simulink model "rm3_ckt_DD_gen_vR2021b"  (R2021b)
settings: Solver=ode4  StartTime=0.0  StopTime=simu.duration  FixedStep=simu.timestep  MaxStep=0.1  MinStep=0.1  RelTol=1e-3
undefined symbols (not defined in the file or in its folder): PTO, R_pto
libraries: fl_lib x22, nesl_utility x19, ee_lib x14
settings Model: Creator=tedbrekken  LastModifiedBy=prana

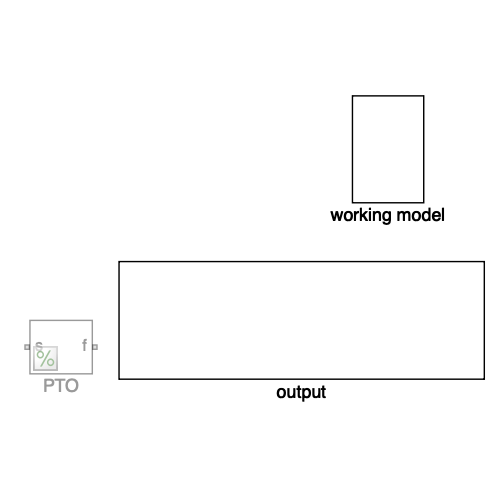
[thumbnail: Simulink's stored preview of the top-level diagram]
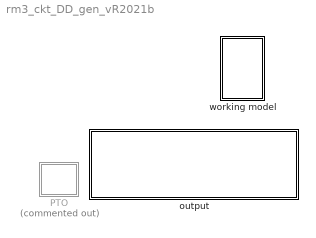
== system rm3_ckt_DD_gen_vR2021b ==
  PTO : Subsystem  Commented=on
  output : Subsystem
  working model : Subsystem

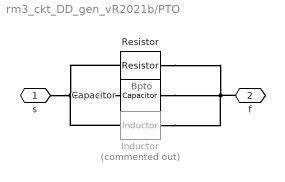
== system rm3_ckt_DD_gen_vR2021b/PTO ==
  note: Bpto
  Capacitor : fl_lib/Electrical/Electrical Elements/Capacitor  c=C_pto F  r=1e-6 Ohm  g=0 1/Ohm  i_specify=off  i_priority=None  i=0 A  i_nominal_specify=off  i_nominal_unit=A  i_nominal_value=1  v_specify=off  v_priority=None  v=0 V  v_nominal_specify=off  v_nominal_unit=V  v_nominal_value=1  vc_specify=off  vc_priority=High  vc=0 V  vc_nominal_specify=off  vc_nominal_unit=V  vc_nominal_value=1
  Inductor : ee_lib/Passive/Inductor  Commented=on  l=L_pto H  L_tol=20  enable_L_tol=0  tol_distribution=1  nSigma=4  r=0 Ohm  g=1e-9 1/Ohm  enable_operating_limits=0  operating_limit_action=2  max_working_current=1 A  power_rating=1 W  enable_faults=0  fault_action=1  lambdaPercent=50  k_faulted=0.9999  turnsShort=0  openCct=0  groundShort=0  groundShortG=0 1/Ohm  tau_fault=1e-3 s  enable_temporal_fault=0  t_fault=1 s  enable_behavioral_fault=0  max_permissible_voltage=100 V  n_fail_on_voltage=1  max_permissible_current=1 A  t_fail_on_current=1 s  i_L_specify=off  i_L_priority=High  i_L=0 A  i_L_nominal_specify=off  i_L_nominal_unit=A  i_L_nominal_value=1
  Resistor : ee_lib/Passive/Resistor  R=R_pto Ohm  R_tol=5  enable_R_tol=0  tol_distribution=1  nSigma=4  enable_operating_limits=0  operating_limit_action=2  max_working_voltage=100 V  power_rating=1 W  enable_faults=0  fault_action=1  R_faulted=inf Ohm  enable_temporal_fault=0  t_fault=1 s  enable_behavioral_fault=0  max_permissible_current=1 A  t_fail_on_current=1 s  noise_mode=0  sample_time=1e-3 s  repeatability=1  auto_seed=3499211588  user_seed=0  Tdevice=25 degC  power_derating_T1=70 degC  power_derating_T2=155 degC  operating_temperature_range_vec=[-50, 150] degC  alpha=3.93e-3 1/K  Tmeas=25 degC  thermal_mass=100 J/K  temperature_specify=off  temperature_priority=High  temperature=298.15 K  temperature_nominal_specify=off  temperature_nominal_unit=K  temperature_nominal_value=1
  s : PMIOPort  Side=Left
  f : PMIOPort  Port=2  Side=Right
  connections:
  s/RConn1 -- Resistor/LConn1 -- Inductor/LConn1 -- Capacitor/LConn1
  f/RConn1 -- Resistor/RConn1 -- Inductor/RConn1 -- Capacitor/RConn1

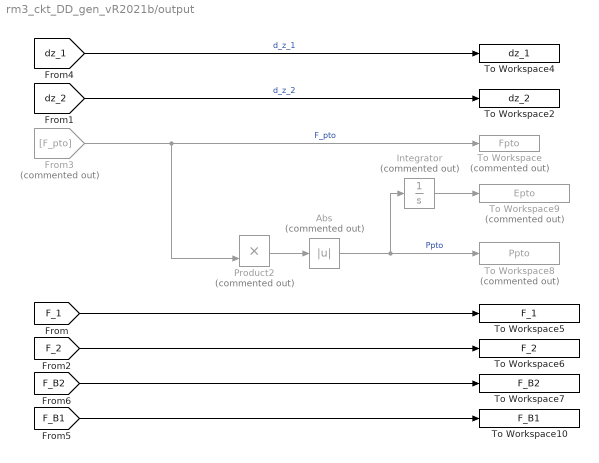
== system rm3_ckt_DD_gen_vR2021b/output ==
  Abs : Abs  Commented=on
  From3 : From  Commented=on  GotoTag=F_pto  TagVisibility=global
  Integrator : Integrator  Commented=on
  Product2 : Product  Commented=on
  To Workspace : ToWorkspace  Commented=on  VariableName=Fpto  SaveFormat=Timeseries  SampleTime=-1
  To Workspace10 : ToWorkspace  VariableName=F_B1  SaveFormat=Timeseries  SampleTime=-1
  To Workspace2 : ToWorkspace  VariableName=dz_2  SaveFormat=Timeseries  SampleTime=-1
  To Workspace4 : ToWorkspace  VariableName=dz_1  SaveFormat=Timeseries  SampleTime=-1
  To Workspace5 : ToWorkspace  VariableName=F_1  SaveFormat=Timeseries  SampleTime=-1
  To Workspace6 : ToWorkspace  VariableName=F_2  SaveFormat=Timeseries  SampleTime=-1
  To Workspace7 : ToWorkspace  VariableName=F_B2  SaveFormat=Timeseries  SampleTime=-1
  To Workspace8 : ToWorkspace  Commented=on  VariableName=Ppto  SaveFormat=Timeseries  SampleTime=-1
  To Workspace9 : ToWorkspace  Commented=on  VariableName=Epto  SaveFormat=Timeseries  SampleTime=-1
  wires:
  Integrator/1 -> To Workspace9/1
  [dz_1] -> To Workspace4/1  "d_z_1"
  From3/1 -> To Workspace/1, Product2/2  "F_pto"
  Abs/1 -> To Workspace8/1, Integrator/1  "Ppto"
  Product2/1 -> Abs/1
  [dz_2] -> To Workspace2/1  "d_z_2"
  [F_1] -> To Workspace5/1
  [F_2] -> To Workspace6/1
  [F_B2] -> To Workspace7/1
  [F_B1] -> To Workspace10/1

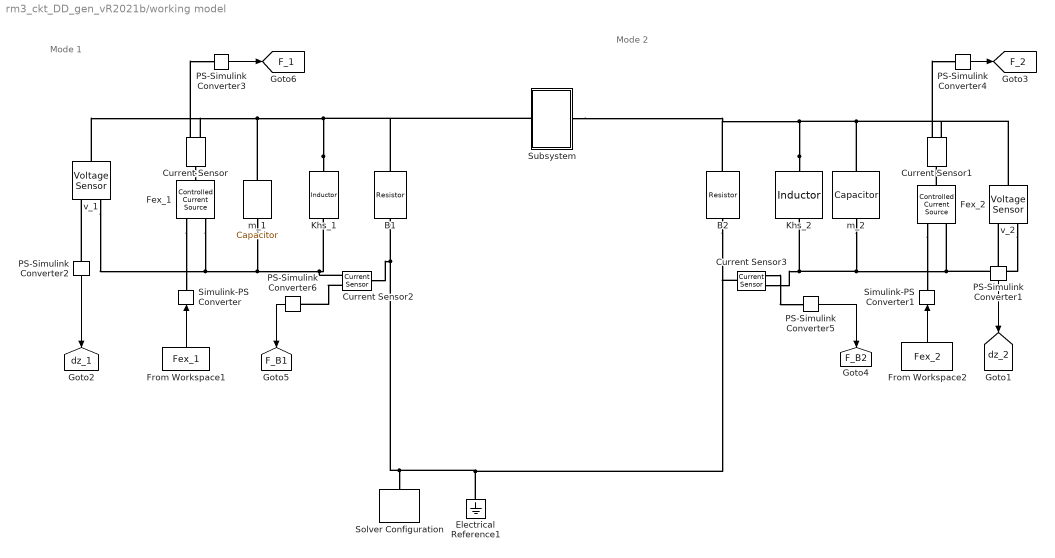
== system rm3_ckt_DD_gen_vR2021b/working model ==
  note: Mode 1
  note: Mode 2
  B1 : ee_lib/Passive/Resistor  R=1/PTO.B_rad22(1,1) Ohm  R_tol=5  enable_R_tol=0  tol_distribution=1  nSigma=4  enable_operating_limits=0  operating_limit_action=2  max_working_voltage=100 V  power_rating=1 W  enable_faults=0  fault_action=1  R_faulted=inf Ohm  enable_temporal_fault=0  t_fault=1 s  enable_behavioral_fault=0  max_permissible_current=1 A  t_fail_on_current=1 s  noise_mode=0  sample_time=1e-3 s  repeatability=1  auto_seed=545404223  user_seed=0  Tdevice=25 degC  power_derating_T1=70 degC  power_derating_T2=155 degC  operating_temperature_range_vec=[-50, 150] degC  alpha=3.93e-3 1/K  Tmeas=25 degC  thermal_mass=100 J/K  temperature_specify=off  temperature_priority=High  temperature=298.15 K  temperature_nominal_specify=off  temperature_nominal_unit=K  temperature_nominal_value=1
  B2 : ee_lib/Passive/Resistor  R=1/PTO.B_rad22(2,2) Ohm  R_tol=5  enable_R_tol=0  tol_distribution=1  nSigma=4  enable_operating_limits=0  operating_limit_action=2  max_working_voltage=100 V  power_rating=1 W  enable_faults=0  fault_action=1  R_faulted=inf Ohm  enable_temporal_fault=0  t_fault=1 s  enable_behavioral_fault=0  max_permissible_current=1 A  t_fail_on_current=1 s  noise_mode=0  sample_time=1e-3 s  repeatability=1  auto_seed=3922919431  user_seed=0  Tdevice=25 degC  power_derating_T1=70 degC  power_derating_T2=155 degC  operating_temperature_range_vec=[-50, 150] degC  alpha=3.93e-3 1/K  Tmeas=25 degC  thermal_mass=100 J/K  temperature_specify=off  temperature_priority=High  temperature=298.15 K  temperature_nominal_specify=off  temperature_nominal_unit=K  temperature_nominal_value=1
  Current Sensor{,1..3} (4 alike) : fl_lib/Electrical/Electrical Sensors/Current Sensor
  Electrical Reference1 : fl_lib/Electrical/Electrical Elements/Electrical Reference
  Fex_1 : fl_lib/Electrical/Electrical Sources/Controlled Current Source
  Fex_2 : fl_lib/Electrical/Electrical Sources/Controlled Current Source
  From Workspace1 : FromWorkspace  VariableName=Fex_1
  From Workspace2 : FromWorkspace  VariableName=Fex_2
  Khs_1 : ee_lib/Passive/Inductor  l=1/PTO.K_hs(1,1) H  L_tol=5  enable_L_tol=0  tol_distribution=1  nSigma=4  r=0 Ohm  g=1e-9 1/Ohm  enable_operating_limits=0  operating_limit_action=2  max_working_current=1 A  power_rating=1 W  enable_faults=0  fault_action=1  lambdaPercent=50  k_faulted=0.9999  turnsShort=0  openCct=0  groundShort=0  groundShortG=0 1/Ohm  tau_fault=1e-3 s  enable_temporal_fault=0  t_fault=1 s  enable_behavioral_fault=0  max_permissible_voltage=100 V  n_fail_on_voltage=1  max_permissible_current=1 A  t_fail_on_current=1 s  i_L_specify=off  i_L_priority=High  i_L=0 A  i_L_nominal_specify=off  i_L_nominal_unit=A  i_L_nominal_value=1
  Khs_2 : ee_lib/Passive/Inductor  l=1/PTO.K_hs(2,2) H  L_tol=5  enable_L_tol=0  tol_distribution=1  nSigma=4  r=0 Ohm  g=1e-9 1/Ohm  enable_operating_limits=0  operating_limit_action=2  max_working_current=1 A  power_rating=1 W  enable_faults=0  fault_action=1  lambdaPercent=50  k_faulted=0.9999  turnsShort=0  openCct=0  groundShort=0  groundShortG=0 1/Ohm  tau_fault=1e-3 s  enable_temporal_fault=0  t_fault=1 s  enable_behavioral_fault=0  max_permissible_voltage=100 V  n_fail_on_voltage=1  max_permissible_current=1 A  t_fail_on_current=1 s  i_L_specify=off  i_L_priority=High  i_L=0 A  i_L_nominal_specify=off  i_L_nominal_unit=A  i_L_nominal_value=1
  PS-Simulink Converter{1..6} (6 alike) : nesl_utility/PS-Simulink Converter  PhysicalDomain=network_engine_domain  SubClassName=ps_output  LeftPortType=input  RightPortType=output  PseudoPeriodic=off  Frequencies=[]  Unit=inherit  AffineConversion=off
      settings: SourceProductBaseCode=PW,SS
  Simulink-PS Converter : nesl_utility/Simulink-PS Converter  PhysicalDomain=network_engine_domain  SubClassName=ps_input  LeftPortType=input  RightPortType=output  PseudoPeriodic=off  Frequencies=[]  NoiseDistribution=none  NoiseParameters=[]  Unit=1  AffineConversion=off  FilteringAndDerivatives=provide  SimscapeFilterOrder=1  InputFilterTimeConstant=0.001  UdotUserProvided=0
      settings: SourceProductBaseCode=PW,SS
  Simulink-PS Converter1 : nesl_utility/Simulink-PS Converter  PhysicalDomain=network_engine_domain  SubClassName=ps_input  LeftPortType=input  RightPortType=output  PseudoPeriodic=off  Frequencies=[]  NoiseDistribution=none  NoiseParameters=[]  Unit=1  AffineConversion=off  FilteringAndDerivatives=provide  SimscapeFilterOrder=1  InputFilterTimeConstant=0.001  UdotUserProvided=0
      settings: SourceProductBaseCode=PW,SS
  Solver Configuration : nesl_utility/Solver Configuration  PhysicalDomain=network_engine_domain  SubClassName=solver  LeftPortType=input  RightPortType=generic  Tones=[]  Harmonics=[]  SimulateNoise=off  Profile=off  UseLocalSampling=off  EnableSwitchedLinearOptims=on  FrequencyDomain=off  UseCCode=off  RelTol=0.001  AbsTol=1e-06  MinStep=1e-09  ToWorkspace=off  RevertToSquareIcSolve=off  NumHomotopyIterations=100  PhasorMode=off  PhasorModeNumHarmonics=1  DoDC=off  ResidualTolerance=1e-09  UseLocalSolver=off  LocalSolverChoice=NE_TRAPEZOIDAL_ADVANCER  LocalSolverSampleTime=0.1  DoFixedCost=off  MaxNonlinIter=3  MaxModeIter=2  ComputeImpulses=off  ImpulseIterations=2  LinearAlgebra=auto  EquationFormulation=NE_TIME_EF  DelaysMemoryBudget=1024  AutomaticFiltering=off  FilteringTimeConstant=0.001  PartitionStorageMethod=AS_NEEDED  PartitionMemoryBudget=1024  PartitionMethod=ROBUST
      settings: SourceProductBaseCode=PW,SS
  Subsystem : Subsystem
  m_1 : ee_lib/Passive/Capacitor  cap_option=0  c=PTO.Mass(1,1) F  Cvec=[1e-05, 1e-06] F  Vvec=[0, 10] V  CV_table_symmetry=1  f_vec=[1, 10] kHz  DFext_vec=[.8, 1.2]  C_tol=5  enable_C_tol=0  tol_distribution=1  nSigma=4  r=0 Ohm  g=0 1/Ohm  averaging_period=0 s  enable_operating_limits=0  operating_limit_action=2  max_working_voltage_range=[-25, 25] V  power_rating=1 W  enable_faults=0  fault_action=1  Cscale_faulted=100  R_faulted=1e-3 Ohm  G_faulted=0 1/Ohm  tau_fault=1e-3 s  enable_temporal_fault=0  t_fault=1 s  enable_behavioral_fault=0  max_permissible_voltage_range=[-100, 100] V  t_fail_on_voltage=1 s  i_specify=off  i_priority=None  i=0 A  i_nominal_specify=off  i_nominal_unit=A  i_nominal_value=1  v_specify=off  v_priority=None  v=0 V  v_nominal_specify=off  v_nominal_unit=V  v_nominal_value=1  vc_specify=off  vc_priority=High  vc=0 V  vc_nominal_specify=off  vc_nominal_unit=V  vc_nominal_value=1
  m_2 : ee_lib/Passive/Capacitor  cap_option=0  c=PTO.Mass(2,2) F  Cvec=[1e-05, 1e-06] F  Vvec=[0, 10] V  CV_table_symmetry=1  f_vec=[1, 10] kHz  DFext_vec=[.8, 1.2]  C_tol=5  enable_C_tol=0  tol_distribution=1  nSigma=4  r=0 Ohm  g=0 1/Ohm  averaging_period=0 s  enable_operating_limits=0  operating_limit_action=2  max_working_voltage_range=[-25, 25] V  power_rating=1 W  enable_faults=0  fault_action=1  Cscale_faulted=100  R_faulted=1e-3 Ohm  G_faulted=0 1/Ohm  tau_fault=1e-3 s  enable_temporal_fault=0  t_fault=1 s  enable_behavioral_fault=0  max_permissible_voltage_range=[-100, 100] V  t_fail_on_voltage=1 s  i_specify=off  i_priority=None  i=0 A  i_nominal_specify=off  i_nominal_unit=A  i_nominal_value=1  v_specify=off  v_priority=None  v=0 V  v_nominal_specify=off  v_nominal_unit=V  v_nominal_value=1  vc_specify=off  vc_priority=High  vc=0 V  vc_nominal_specify=off  vc_nominal_unit=V  vc_nominal_value=1
  v_1 : fl_lib/Electrical/Electrical Sensors/Voltage Sensor
  v_2 : fl_lib/Electrical/Electrical Sensors/Voltage Sensor
  tag scope: F_1=global, F_2=global, F_B1=global, F_B2=global, dz_1=global, dz_2=global
  wires:
  From Workspace1/1 -> Simulink-PS Converter/1
  PS-Simulink Converter3/1 -> [F_1]
  PS-Simulink Converter2/1 -> [dz_1]
  From Workspace2/1 -> Simulink-PS Converter1/1
  PS-Simulink Converter4/1 -> [F_2]
  PS-Simulink Converter1/1 -> [dz_2]
  PS-Simulink Converter5/1 -> [F_B2]
  PS-Simulink Converter6/1 -> [F_B1]
  connections:
  Fex_2/LConn1 -- Current Sensor1/LConn1
  Current Sensor/LConn1 -- Fex_1/LConn1
  Fex_2/RConn1 -- Simulink-PS Converter1/RConn1
  PS-Simulink Converter1/LConn1 -- v_2/RConn1
  Khs_1/LConn1 -- B1/LConn1 -- Subsystem/LConn1 -- Current Sensor/RConn2 -- v_1/LConn1 -- m_1/LConn1
  Fex_1/RConn1 -- Simulink-PS Converter/RConn1
  PS-Simulink Converter2/LConn1 -- v_1/RConn1
  m_2/RConn1 -- Current Sensor3/RConn2 -- Khs_2/RConn1 -- v_2/RConn2 -- Fex_2/RConn2
  Current Sensor1/RConn1 -- PS-Simulink Converter4/LConn1
  Current Sensor/RConn1 -- PS-Simulink Converter3/LConn1
  Khs_2/LConn1 -- B2/LConn1 -- Subsystem/RConn1 -- v_2/LConn1 -- Current Sensor1/RConn2 -- m_2/LConn1
  Fex_1/RConn2 -- Current Sensor2/RConn2 -- Khs_1/RConn1 -- m_1/RConn1 -- v_1/RConn2
  Electrical Reference1/LConn1 -- Current Sensor3/LConn1 -- B2/RConn1 -- B1/RConn1 -- Current Sensor2/LConn1 -- Solver Configuration/RConn1
  Current Sensor2/RConn1 -- PS-Simulink Converter6/LConn1
  Current Sensor3/RConn1 -- PS-Simulink Converter5/LConn1

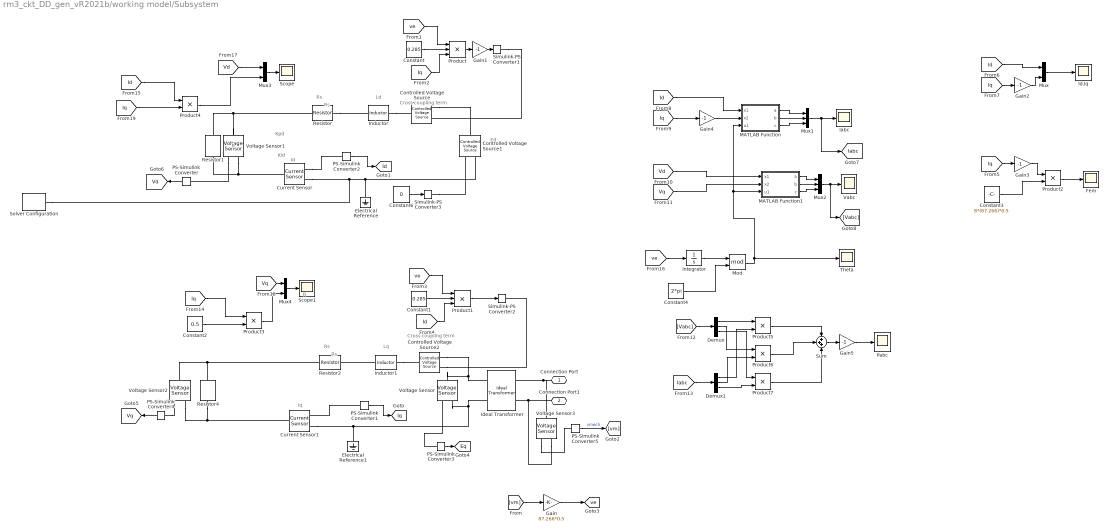
== system rm3_ckt_DD_gen_vR2021b/working model/Subsystem ==
  note: Iq
  note: Id
  note: R
  note: Cross coupling term
  note: Ld
  note: Rs
  note: Ed
  note: Rs
  note: Cross coupling term
  note: R
  note: Lq
  note: Rs
  note: Rs
  note: Kpd
  note: Kid
  Constant : Constant  Value=0.285
  Constant1 : Constant  Value=0.285
  Constant2 : Constant  Value=0.5
  Constant3 : Constant  Value=8*(87.266)*0.5
  Constant4 : Constant  Value=2*pi
  Constant6 : Constant  Value=0
  Controlled Voltage Source : fl_lib/Electrical/Electrical Sources/Controlled Voltage Source
  Controlled Voltage Source1 : fl_lib/Electrical/Electrical Sources/Controlled Voltage Source
  Controlled Voltage Source2 : fl_lib/Electrical/Electrical Sources/Controlled Voltage Source
  Current Sensor : fl_lib/Electrical/Electrical Sensors/Current Sensor
  Current Sensor1 : fl_lib/Electrical/Electrical Sensors/Current Sensor
  Demux : Demux  Outputs=3
  Demux1 : Demux  Outputs=3
  Electrical Reference : fl_lib/Electrical/Electrical Elements/Electrical Reference
  Electrical Reference1 : fl_lib/Electrical/Electrical Elements/Electrical Reference
  Fem : Scope
  Gain : Gain  Gain=87.266*0.5
  Gain{1..5} (5 alike) : Gain  Gain=-1
  Iabc : Scope
  Id,Iq : Scope
  Ideal Transformer : fl_lib/Electrical/Electrical Elements/Ideal Transformer  n=8*(87.266)*0.5  i1_specify=off  i1_priority=None  i1=0 A  i1_nominal_specify=off  i1_nominal_unit=A  i1_nominal_value=1  v1_specify=off  v1_priority=None  v1=0 V  v1_nominal_specify=off  v1_nominal_unit=V  v1_nominal_value=1  i2_specify=off  i2_priority=None  i2=0 A  i2_nominal_specify=off  i2_nominal_unit=A  i2_nominal_value=1  v2_specify=off  v2_priority=None  v2=0 V  v2_nominal_specify=off  v2_nominal_unit=V  v2_nominal_value=1
      settings: SourceProductBaseCode=SS
  Inductor : ee_lib/Passive/Inductor  l=0.285 H  L_tol=20  enable_L_tol=0  tol_distribution=1  nSigma=4  r=0 Ohm  g=0 1/Ohm  enable_operating_limits=0  operating_limit_action=2  max_working_current=1 A  power_rating=1 W  enable_faults=0  fault_action=1  lambdaPercent=50  k_faulted=0.9999  turnsShort=0  openCct=0  groundShort=0  groundShortG=0 1/Ohm  tau_fault=1e-3 s  enable_temporal_fault=0  t_fault=1 s  enable_behavioral_fault=0  max_permissible_voltage=100 V  n_fail_on_voltage=1  max_permissible_current=1 A  t_fail_on_current=1 s  i_L_specify=off  i_L_priority=High  i_L=0 A  i_L_nominal_specify=off  i_L_nominal_unit=A  i_L_nominal_value=1
  Inductor1 : ee_lib/Passive/Inductor  l=0.285 H  L_tol=20  enable_L_tol=0  tol_distribution=1  nSigma=4  r=0 Ohm  g=0 1/Ohm  enable_operating_limits=0  operating_limit_action=2  max_working_current=1 A  power_rating=1 W  enable_faults=0  fault_action=1  lambdaPercent=50  k_faulted=0.9999  turnsShort=0  openCct=0  groundShort=0  groundShortG=0 1/Ohm  tau_fault=1e-3 s  enable_temporal_fault=0  t_fault=1 s  enable_behavioral_fault=0  max_permissible_voltage=100 V  n_fail_on_voltage=1  max_permissible_current=1 A  t_fail_on_current=1 s  i_L_specify=off  i_L_priority=High  i_L=0 A  i_L_nominal_specify=off  i_L_nominal_unit=A  i_L_nominal_value=1
  Integrator : Integrator
  MATLAB Function : MATLAB Function  TreatAsAtomicUnit=on
  MATLAB Function1 : MATLAB Function  TreatAsAtomicUnit=on
  Mod : Math  Operator=mod  SaturateOnIntegerOverflow=on
  Mux : Mux  Inputs=2
  Mux1 : Mux  Inputs=3
  Mux2 : Mux  Inputs=3
  Mux3 : Mux  Inputs=2
  Mux4 : Mux  Inputs=2
  PS-Simulink Converter{,1..5} (6 alike) : nesl_utility/PS-Simulink Converter  PhysicalDomain=network_engine_domain  SubClassName=ps_output  LeftPortType=input  RightPortType=output  PseudoPeriodic=off  Frequencies=[]  Unit=inherit  AffineConversion=off
      settings: SourceProductBaseCode=PW,SS
  Pabc : Scope
  Product : Product  Inputs=3
  Product1 : Product  Inputs=3
  Product{2..7} (6 alike) : Product
  Resistor : ee_lib/Passive/Resistor  R=4.58 Ohm  R_tol=5  enable_R_tol=0  tol_distribution=1  nSigma=4  enable_operating_limits=0  operating_limit_action=2  max_working_voltage=100 V  power_rating=1 W  enable_faults=0  fault_action=1  R_faulted=inf Ohm  enable_temporal_fault=0  t_fault=1 s  enable_behavioral_fault=0  max_permissible_current=1 A  t_fail_on_current=1 s  noise_mode=0  sample_time=1e-3 s  repeatability=1  auto_seed=1684602222  user_seed=0  Tdevice=25 degC  power_derating_T1=70 degC  power_derating_T2=155 degC  operating_temperature_range_vec=[-50, 150] degC  alpha=3.93e-3 1/K  Tmeas=25 degC  thermal_mass=100 J/K  temperature_specify=off  temperature_priority=High  temperature=298.15 K  temperature_nominal_specify=off  temperature_nominal_unit=K  temperature_nominal_value=1
  Resistor1 : ee_lib/Passive/Resistor  R=0.5 Ohm  R_tol=5  enable_R_tol=0  tol_distribution=1  nSigma=4  enable_operating_limits=0  operating_limit_action=2  max_working_voltage=100 V  power_rating=1 W  enable_faults=0  fault_action=1  R_faulted=inf Ohm  enable_temporal_fault=0  t_fault=1 s  enable_behavioral_fault=0  max_permissible_current=1 A  t_fail_on_current=1 s  noise_mode=0  sample_time=1e-3 s  repeatability=1  auto_seed=2815256101  user_seed=0  Tdevice=25 degC  power_derating_T1=70 degC  power_derating_T2=155 degC  operating_temperature_range_vec=[-50, 150] degC  alpha=3.93e-3 1/K  Tmeas=25 degC  thermal_mass=100 J/K  temperature_specify=off  temperature_priority=High  temperature=298.15 K  temperature_nominal_specify=off  temperature_nominal_unit=K  temperature_nominal_value=1
  Resistor2 : ee_lib/Passive/Resistor  R=4.58 Ohm  R_tol=5  enable_R_tol=0  tol_distribution=1  nSigma=4  enable_operating_limits=0  operating_limit_action=2  max_working_voltage=100 V  power_rating=1 W  enable_faults=0  fault_action=1  R_faulted=inf Ohm  enable_temporal_fault=0  t_fault=1 s  enable_behavioral_fault=0  max_permissible_current=1 A  t_fail_on_current=1 s  noise_mode=0  sample_time=1e-3 s  repeatability=1  auto_seed=735241226  user_seed=0  Tdevice=25 degC  power_derating_T1=70 degC  power_derating_T2=155 degC  operating_temperature_range_vec=[-50, 150] degC  alpha=3.93e-3 1/K  Tmeas=25 degC  thermal_mass=100 J/K  temperature_specify=off  temperature_priority=High  temperature=298.15 K  temperature_nominal_specify=off  temperature_nominal_unit=K  temperature_nominal_value=1
  Resistor4 : ee_lib/Passive/Resistor  R=0.5 Ohm  R_tol=5  enable_R_tol=0  tol_distribution=1  nSigma=4  enable_operating_limits=0  operating_limit_action=2  max_working_voltage=100 V  power_rating=1 W  enable_faults=0  fault_action=1  R_faulted=inf Ohm  enable_temporal_fault=0  t_fault=1 s  enable_behavioral_fault=0  max_permissible_current=1 A  t_fail_on_current=1 s  noise_mode=0  sample_time=1e-3 s  repeatability=1  auto_seed=1822504018  user_seed=0  Tdevice=25 degC  power_derating_T1=70 degC  power_derating_T2=155 degC  operating_temperature_range_vec=[-50, 150] degC  alpha=3.93e-3 1/K  Tmeas=25 degC  thermal_mass=100 J/K  temperature_specify=off  temperature_priority=High  temperature=298.15 K  temperature_nominal_specify=off  temperature_nominal_unit=K  temperature_nominal_value=1
  Scope : Scope
  Scope1 : Scope
  Simulink-PS Converter1 : nesl_utility/Simulink-PS Converter  PhysicalDomain=network_engine_domain  SubClassName=ps_input  LeftPortType=input  RightPortType=output  PseudoPeriodic=off  Frequencies=[]  NoiseDistribution=none  NoiseParameters=[]  Unit=1  AffineConversion=off  FilteringAndDerivatives=provide  SimscapeFilterOrder=1  InputFilterTimeConstant=0.001  UdotUserProvided=0
      settings: SourceProductBaseCode=PW,SS
  Simulink-PS Converter2 : nesl_utility/Simulink-PS Converter  PhysicalDomain=network_engine_domain  SubClassName=ps_input  LeftPortType=input  RightPortType=output  PseudoPeriodic=off  Frequencies=[]  NoiseDistribution=none  NoiseParameters=[]  Unit=1  AffineConversion=off  FilteringAndDerivatives=provide  SimscapeFilterOrder=1  InputFilterTimeConstant=0.001  UdotUserProvided=0
      settings: SourceProductBaseCode=PW,SS
  Simulink-PS Converter3 : nesl_utility/Simulink-PS Converter  PhysicalDomain=network_engine_domain  SubClassName=ps_input  LeftPortType=input  RightPortType=output  PseudoPeriodic=off  Frequencies=[]  NoiseDistribution=none  NoiseParameters=[]  Unit=1  AffineConversion=off  FilteringAndDerivatives=provide  SimscapeFilterOrder=1  InputFilterTimeConstant=0.001  UdotUserProvided=0
      settings: SourceProductBaseCode=PW,SS
  Solver Configuration : nesl_utility/Solver Configuration  PhysicalDomain=network_engine_domain  SubClassName=solver  LeftPortType=input  RightPortType=generic  Tones=[]  Harmonics=[]  SimulateNoise=off  Profile=off  UseLocalSampling=off  EnableSwitchedLinearOptims=on  FrequencyDomain=off  UseCCode=off  RelTol=0.001  AbsTol=1e-06  MinStep=1e-09  ToWorkspace=off  RevertToSquareIcSolve=off  NumHomotopyIterations=100  PhasorMode=off  PhasorModeNumHarmonics=1  DoDC=on  ResidualTolerance=1e-09  UseLocalSolver=off  LocalSolverChoice=NE_BACKWARD_EULER_ADVANCER  LocalSolverSampleTime=0.001  DoFixedCost=off  MaxNonlinIter=3  MaxModeIter=2  ComputeImpulses=off  ImpulseIterations=2  LinearAlgebra=auto  EquationFormulation=NE_TIME_EF  DelaysMemoryBudget=1024  AutomaticFiltering=off  FilteringTimeConstant=0.001  PartitionStorageMethod=AS_NEEDED  PartitionMemoryBudget=1024  PartitionMethod=ROBUST
      settings: SourceProductBaseCode=PW,SS
  Sum : Sum  Inputs=+++
  Theta : Scope
  Vabc : Scope
  Voltage Sensor{,1..3} (4 alike) : fl_lib/Electrical/Electrical Sensors/Voltage Sensor
  Connection Port : PMIOPort  Side=Left
  Connection Port1 : PMIOPort  Port=2  Side=Right
  tag scope: Eq=global, Iabc=global, Id=global, Iq=global, Vd=global, Vq=global, ve=global
  wires:
  PS-Simulink Converter1/1 -> [Iq]
  Constant4/1 -> Mod/2
  [Id] -> MATLAB Function/1(x1)
  Product4/1 -> Mux3/2
  Demux/2 -> Product6/1
  Mux4/1 -> Scope1/1
  [ve] -> Product1/1
  [Vd] -> Mux3/1
  [Vq] -> Mux4/1
  [Vq] -> MATLAB Function1/2(x2)
  [Iq] -> Product4/2
  Sum/1 -> Gain5/1
  Demux/1 -> Product5/1
  [ve] -> Product/1
  PS-Simulink Converter2/1 -> [Id]
  Product2/1 -> Fem/1
  [ve] -> Integrator/1
  [Id] -> Product1/3
  Mux/1 -> Id,Iq/1
  [Iq] -> Gain4/1
  [Id] -> Product4/1
  Constant6/1 -> Simulink-PS Converter3/1
  [Iq] -> Gain3/1
  Product6/1 -> Sum/2
  Gain2/1 -> Mux/2
  Constant3/1 -> Product2/2
  Demux/3 -> Product7/1
  PS-Simulink Converter3/1 -> [Eq]
  [Iq] -> Product3/1
  [Iq] -> Gain2/1
  Mux3/1 -> Scope/1
  [Id] -> Mux/1
  Constant/1 -> Product/2
  Constant2/1 -> Product3/2
  [vm] -> Gain/1
  Demux1/3 -> Product7/2
  Mux1/1 -> [Iabc], Iabc/1
  [Iq] -> Product/3
  PS-Simulink Converter/1 -> [Vd]
  Product5/1 -> Sum/1
  Product1/1 -> Simulink-PS Converter2/1
  Demux1/2 -> Product6/2
  Demux1/1 -> Product5/2
  MATLAB Function/3(c) -> Mux1/3
  Mod/1 -> MATLAB Function1/3(u1), MATLAB Function/3(u1), Theta/1
  Integrator/1 -> Mod/1
  [Iabc] -> Demux1/1
  Product7/1 -> Sum/3
  Gain5/1 -> Pabc/1
  Product3/1 -> Mux4/2
  [Vd] -> MATLAB Function1/1(x1)
  Gain3/1 -> Product2/1
  Gain1/1 -> Simulink-PS Converter1/1
  Gain/1 -> [ve]
  MATLAB Function1/3(c) -> Mux2/3
  [Vabc] -> Demux/1
  Constant1/1 -> Product1/2
  MATLAB Function/1(a) -> Mux1/1
  MATLAB Function1/2(b) -> Mux2/2
  MATLAB Function/2(b) -> Mux1/2
  MATLAB Function1/1(a) -> Mux2/1
  Mux2/1 -> [Vabc], Vabc/1
  Product/1 -> Gain1/1
  Gain4/1 -> MATLAB Function/2(x2)
  PS-Simulink Converter5/1 -> [vm]  "vmech"
  PS-Simulink Converter4/1 -> [Vq]
  connections:
  Simulink-PS Converter1/RConn1 -- Controlled Voltage Source/RConn1
  Current Sensor/RConn1 -- PS-Simulink Converter2/LConn1
  Simulink-PS Converter3/RConn1 -- Controlled Voltage Source1/RConn1
  Resistor2/LConn1 -- Resistor4/LConn1 -- Voltage Sensor2/LConn1
  Resistor/RConn1 -- Inductor/LConn1
  PS-Simulink Converter1/LConn1 -- Current Sensor1/RConn1
  Current Sensor1/LConn1 -- Resistor4/RConn1 -- Voltage Sensor2/RConn2
  Controlled Voltage Source2/RConn2 -- Voltage Sensor/LConn1 -- Ideal Transformer/LConn1
  Current Sensor1/RConn2 -- Electrical Reference1/LConn1 -- Voltage Sensor/RConn2 -- Ideal Transformer/LConn2
  PS-Simulink Converter3/LConn1 -- Voltage Sensor/RConn1
  Voltage Sensor1/RConn1 -- PS-Simulink Converter/LConn1
  Controlled Voltage Source/RConn2 -- Controlled Voltage Source1/LConn1
  Inductor1/RConn1 -- Controlled Voltage Source2/LConn1
  Inductor/RConn1 -- Controlled Voltage Source/LConn1
  Controlled Voltage Source2/RConn1 -- Simulink-PS Converter2/RConn1
  Current Sensor/LConn1 -- Resistor1/RConn1 -- Voltage Sensor1/RConn2
  Inductor1/LConn1 -- Resistor2/RConn1
  Resistor/LConn1 -- Voltage Sensor1/LConn1 -- Resistor1/LConn1
  Connection Port/RConn1 -- Ideal Transformer/RConn1 -- Voltage Sensor3/LConn1
  Voltage Sensor3/RConn1 -- PS-Simulink Converter5/LConn1
  Electrical Reference/LConn1 -- Solver Configuration/RConn1 -- Current Sensor/RConn2 -- Controlled Voltage Source1/RConn2
  PS-Simulink Converter4/LConn1 -- Voltage Sensor2/RConn1
  Voltage Sensor3/RConn2 -- Connection Port1/RConn1 -- Ideal Transformer/RConn2

== matlab function rm3_ckt_DD_gen_vR2021b/working model/Subsystem/MATLAB Function1 ==
  data: x1 input; a output; x2 input; u1 input; b output; c output
function [a,b,c] = fcn(x1,x2,u1)
a = sqrt(2/3)*(sin(u1+pi/2)*(x1) + cos(u1+pi/2)*(x2))
b = sqrt(2/3)*(sin(u1 - (2*pi/3) +pi/2)*(x1) + cos(u1 - (2*pi/3) +pi/2)*(x2))
c = sqrt(2/3)*(sin(u1 + (2*pi/3) +pi/2)*(x1) + cos(u1 + (2*pi/3) +pi/2)*(x2))

== matlab function rm3_ckt_DD_gen_vR2021b/working model/Subsystem/MATLAB Function ==
  data: x1 input; a output; x2 input; u1 input; b output; c output
function [a,b,c] = fcn(x1,x2,u1)
a = sqrt(2/3)*(sin(u1+pi/2)*(x1) + cos(u1+pi/2)*(x2))
b = sqrt(2/3)*(sin(u1 - (2*pi/3) +pi/2)*(x1) + cos(u1 - (2*pi/3) +pi/2)*(x2))
c = sqrt(2/3)*(sin(u1 + (2*pi/3) +pi/2)*(x1) + cos(u1 + (2*pi/3) +pi/2)*(x2))
